simulink model "airbus300_zeitkonstanten"  (R2024a)
settings: Solver=VariableStepAuto  StartTime=0.0  StopTime=10.0  RelTol=1e-3
settings Model: Creator=cunis  LastModifiedBy=cunis

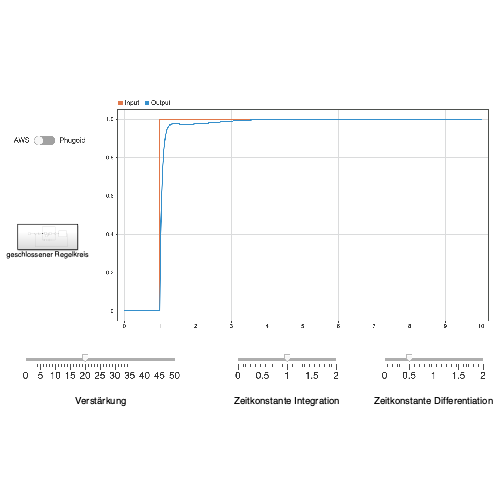
[thumbnail: Simulink's stored preview of the top-level diagram]
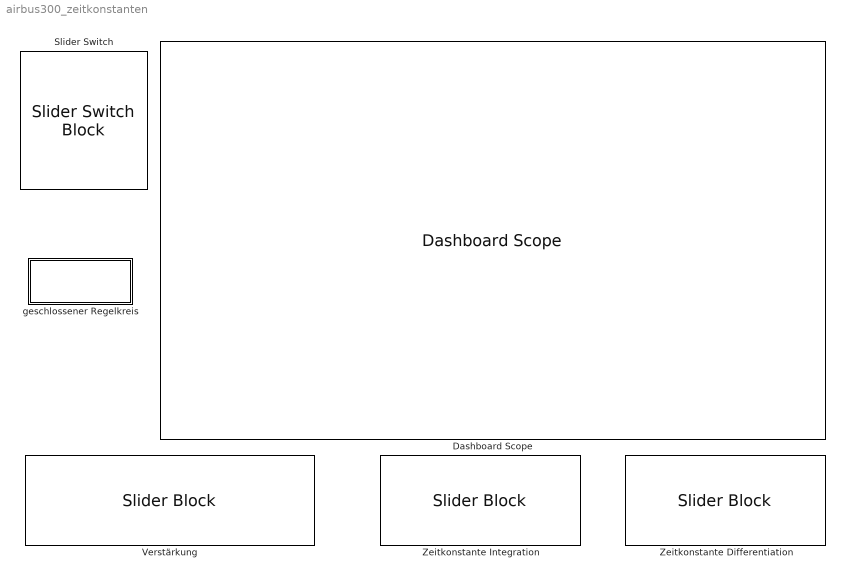
== system airbus300_zeitkonstanten ==
  Dashboard Scope : DashboardScope
  Slider Switch : SliderSwitchBlock  LabelPosition=Hide
      settings: Values={{'AWS', 'Phugoid'}, [1 -1]}
  Verstärkung : SliderBlock  LabelPosition=Hide  ScaleMax=50
  Zeitkonstante Differentiation : SliderBlock  LabelPosition=Hide  ScaleMax=2  TickInterval=0.5
  Zeitkonstante Integration : SliderBlock  LabelPosition=Hide  ScaleMax=2  TickInterval=0.5
  geschlossener Regelkreis : Subsystem

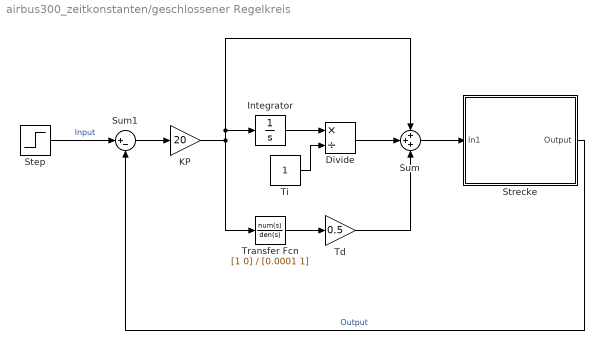
== system airbus300_zeitkonstanten/geschlossener Regelkreis ==
  Divide : Product  Inputs=*/
  Integrator : Integrator
  KP : Gain  Gain=20
  Step : Step  SampleTime=0
  Strecke : Subsystem
  Sum : Sum  Inputs=+++
  Sum1 : Sum  Inputs=|+-
  Td : Gain  Gain=0.5
  Ti : Constant
  Transfer Fcn : TransferFcn  Numerator=[1 0]  Denominator=[0.0001 1]
  wires:
  Sum1/1 -> KP/1
  Divide/1 -> Sum/2
  Integrator/1 -> Divide/1
  Transfer Fcn/1 -> Td/1
  Td/1 -> Sum/3
  Step/1 -> Sum1/1  "Input"
  Sum/1 -> Strecke/1(In1)
  Strecke/1(Output) -> Sum1/2  "Output"
  KP/1 -> Sum/1, Integrator/1, Transfer Fcn/1
  Ti/1 -> Divide/2

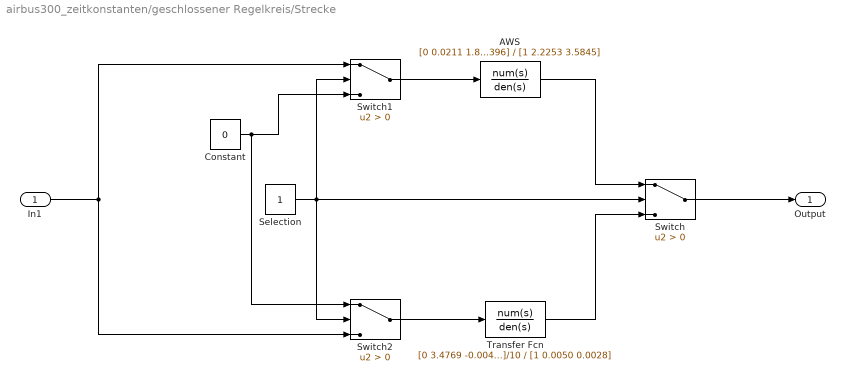
== system airbus300_zeitkonstanten/geschlossener Regelkreis/Strecke ==
  In1 : Inport
  AWS : TransferFcn  Numerator=[0 0.0211 1.8396]  Denominator=[1 2.2253 3.5845]
  Constant : Constant  Value=0
  Selection : Constant
  Switch : Switch  Criteria=u2 > Threshold  SaturateOnIntegerOverflow=off  InputSameDT=off
  Switch1 : Switch  Criteria=u2 > Threshold  SaturateOnIntegerOverflow=off  InputSameDT=off
  Switch2 : Switch  Criteria=u2 > Threshold  SaturateOnIntegerOverflow=off  InputSameDT=off
  Transfer Fcn : TransferFcn  Numerator=[0 3.4769 -0.0049]/10  Denominator=[1 0.0050 0.0028]
  Output : Outport
  wires:
  Switch/1 -> Output/1
  In1/1 -> Switch2/3, Switch1/1
  Selection/1 -> Switch2/2, Switch/2, Switch1/2
  AWS/1 -> Switch/1
  Transfer Fcn/1 -> Switch/3
  Switch1/1 -> AWS/1
  Switch2/1 -> Transfer Fcn/1
  Constant/1 -> Switch2/1, Switch1/3
